simulink model "hw1_1"  (R2014a)
settings: Solver=ode45  StartTime=0.0  StopTime=30  RelTol=1e-3
settings Model: Creator=立宇  LastModifiedBy=立宇

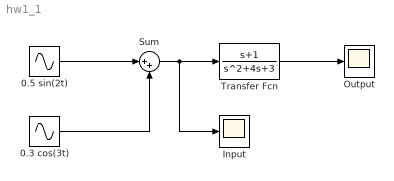
== system hw1_1 ==
  0.3 cos(3t) : Sin  Amplitude=0.3  Frequency=3  SampleTime=0
  0.5 sin(2t) : Sin  Amplitude=0.5  Frequency=2  SampleTime=0
  Input : Scope
  Output : Scope
  Sum : Sum  Inputs=|++
  Transfer Fcn : TransferFcn  Numerator=[1 1]  Denominator=[1 4 3]
  wires:
  0.3 cos(3t)/1 -> Sum/2
  0.5 sin(2t)/1 -> Sum/1
  Transfer Fcn/1 -> Output/1
  Sum/1 -> Transfer Fcn/1, Input/1
